simulink model "unipolar_rz"  (Simulink 7.9)
settings: Solver=ode5  SolverMode=SingleTasking  StartTime=0.0  StopTime=1  FixedStep=1/fs  RelTol=1e-3  AbsTol=1e-6
PreLoadFcn:
  | R=1000; fs=10*R;
undefined symbols (not defined in the file or in its folder): bessel_den, bessel_num
libraries: commnoisgen2 x1, commrandsrc2 x1
settings Model: Creator=amoura  LastModifiedBy=amoura_2
settings DataIOCC: LimitDataPoints=off  SignalLoggingName=sigsOut
settings OptimizationCC: BooleanDataType=off  InitFltsAndDblsToZero=on
settings DebuggingCC: SaveWithParameterizedLinksMsg=none  SignalResolutionControl=TryResolveAllWithWarning  SolverPrmCheckMsg=none  MultiTaskDSMMsg=warning  MultiTaskCondExecSysMsg=none  FcnCallInpInsideContextMsg=Use local settings  StrictBusMsg=None
settings HardwareCC: TargetUnknown=on
settings RTWCC: TemplateMakefile=grt_unix.tmf  IncludeERTFirstTime=on
settings GRTTargetCC: TargetFcnLib=ansi_tfl_tmw.mat  ModelReferenceCompliant=off  CombineOutputUpdateFcns=off  MatFileLogging=off  GRTInterface=on

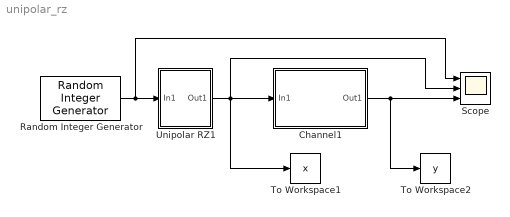
== system unipolar_rz ==
  Channel1 : Subsystem  mask(Communications channel){gain=1, bw=4000, noise_pwr=.01, noise_seed=123}
      mask prompts: bw "Bandwidth (Hz):"; noise_pwr "Noise power:"; noise_seed "Noise seed:"
      mask init:
      | [bessel_num, bessel_den]=besself(8,2*pi*bw);
      | if noise_pwr==0 , noise_var=1e-20; else noise_var=noise_pwr; end
      mask Display: disp('Communications\nchannel')
  Random Integer Generator : commrandsrc2/Random Integer Generator  mul=2  seed=37  Ts=1/R  frameBased=off  sampPerFrame=1  orient=on  outDataType=double
  Scope : Scope  NumInputPorts=3
      settings: TickLabels=on  TimeRange=0.01  YMin=-2~-2~-5  YMax=2~2~5
  To Workspace1 : ToWorkspace  VariableName=x  SampleTime=1/fs
  To Workspace2 : ToWorkspace  VariableName=y  SampleTime=1/fs
  Unipolar RZ1 : Subsystem  mask(Unipolar RZ){Ts=1/R}
      mask prompts: Ts "Smple time (sec):"
      mask help:
      | This block encodes a unipolar NRZ signal into the unipolar RZ (return-to-zero) line code.
      |
      | The output values are +1 during the first half of a nonzero input and  zero otherwise.
      mask Help:
      | This block encodes a unipolar NRZ signal into the unipolar RZ (return-to-zero) line code.
      | 
      | The output values are +1 during the first half of a nonzero input and  zero otherwise.
      mask Display: disp('Unipolar\nRZ')
  wires:
  Random Integer Generator/1 -> Unipolar RZ1/1(In1), Scope/1
  Unipolar RZ1/1(Out1) -> To Workspace1/1, Channel1/1(In1), Scope/2
  Channel1/1(Out1) -> To Workspace2/1, Scope/3

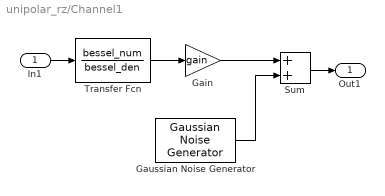
== system unipolar_rz/Channel1 ==
  In1 : Inport
  Gain : Gain  Gain=gain  SaturateOnIntegerOverflow=on  OutDataTypeStr=Inherit: Same as input  ParamDataTypeStr=Inherit: Same as input
  Gaussian Noise Generator : commnoisgen2/Gaussian Noise Generator  m=0  d=noise_pwr  s=noise_seed  Ts=1/fs  frameBased=off  sampPerFrame=1  orient=on  outDataType=double
  Sum : Sum  SaturateOnIntegerOverflow=on  InputSameDT=on  OutDataTypeStr=Inherit: Same as first input
  Transfer Fcn : TransferFcn  Numerator=bessel_num  Denominator=bessel_den
  Out1 : Outport
  wires:
  Gaussian Noise Generator/1 -> Sum/2
  Gain/1 -> Sum/1
  Transfer Fcn/1 -> Gain/1
  In1/1 -> Transfer Fcn/1
  Sum/1 -> Out1/1

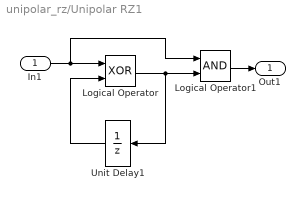
== system unipolar_rz/Unipolar RZ1 ==
  In1 : Inport
  Logical Operator : Logic  Operator=XOR
  Logical Operator1 : Logic
  Unit Delay1 : UnitDelay  SampleTime=Ts/2
  Out1 : Outport
  wires:
  Logical Operator1/1 -> Out1/1
  In1/1 -> Logical Operator1/1, Logical Operator/1
  Logical Operator/1 -> Unit Delay1/1, Logical Operator1/2
  Unit Delay1/1 -> Logical Operator/2
